simulink model "Q2part5"  (R2018b)
settings: Solver=VariableStepAuto  StartTime=0.0  StopTime=5  RelTol=1e-3
values from neighbouring files (symbols this model uses):
  A = [0           1                 0                          0 ... (first row only)    [Q2.m]
  B1 = [0 1/m1 0 1/m1+1/m2]'    [Q2.m]
  B2 = [0                 0 ... (first row only)    [Q2.m]
  C = [0 0 1 0]    [Q2.m]
  l = L'    [Q2.m]
settings Model: Creator=Asus  LastModifiedBy=Asus

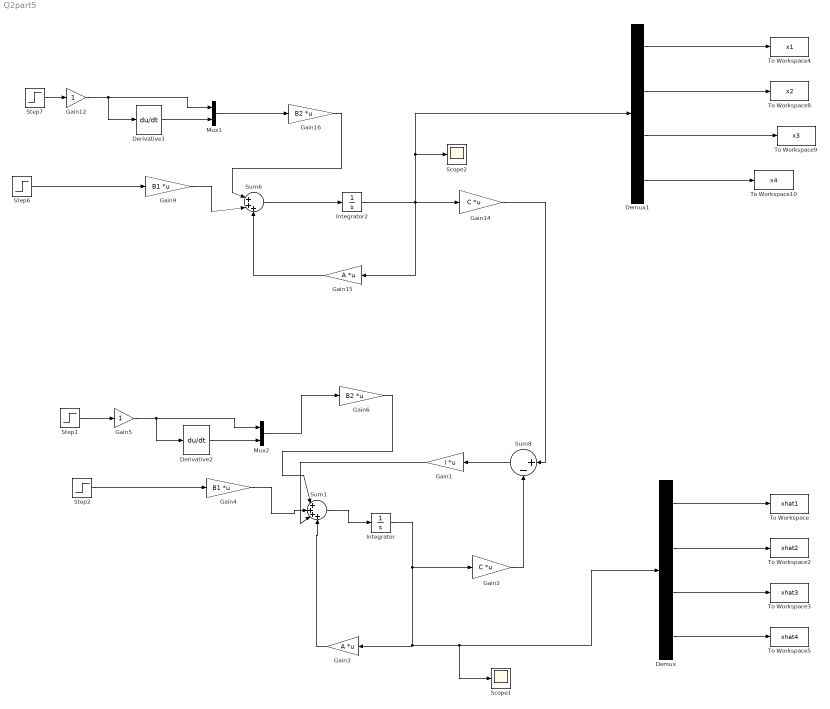
== system Q2part5 ==
  Demux : Demux
  Demux1 : Demux
  Derivative1 : Derivative
  Derivative2 : Derivative
  Gain1 : Gain  Gain=l  Multiplication=Matrix(K*u)
  Gain12 : Gain
  Gain14 : Gain  Gain=C  Multiplication=Matrix(K*u)
  Gain15 : Gain  Gain=A  Multiplication=Matrix(K*u)
  Gain16 : Gain  Gain=B2  Multiplication=Matrix(K*u)
  Gain2 : Gain  Gain=C  Multiplication=Matrix(K*u)
  Gain3 : Gain  Gain=A  Multiplication=Matrix(K*u)
  Gain4 : Gain  Gain=B1  Multiplication=Matrix(K*u)
  Gain5 : Gain
  Gain6 : Gain  Gain=B2  Multiplication=Matrix(K*u)
  Gain9 : Gain  Gain=B1  Multiplication=Matrix(K*u)
  Integrator : Integrator  InitialCondition=[0.5 0 0 0]
  Integrator2 : Integrator
  Mux1 : Mux  Inputs=2
  Mux2 : Mux  Inputs=2
  Scope1 : Scope
  Scope2 : Scope
  Step1 : Step  Time=0  After=0.25  SampleTime=0
  Step2 : Step  Time=0  After=0  SampleTime=0
  Step6 : Step  Time=0  After=0  SampleTime=0
  Step7 : Step  Time=0  After=0.25  SampleTime=0
  Sum1 : Sum  Inputs=|++++
  Sum6 : Sum  Inputs=|+++
  Sum8 : Sum  Inputs=|+-
  To Workspace : ToWorkspace  VariableName=xhat1  SaveFormat=Timeseries  SampleTime=-1
  To Workspace10 : ToWorkspace  VariableName=x4  SaveFormat=Timeseries  SampleTime=-1
  To Workspace2 : ToWorkspace  VariableName=xhat2  SaveFormat=Timeseries  SampleTime=-1
  To Workspace3 : ToWorkspace  VariableName=xhat3  SaveFormat=Timeseries  SampleTime=-1
  To Workspace4 : ToWorkspace  VariableName=x1  SaveFormat=Timeseries  SampleTime=-1
  To Workspace5 : ToWorkspace  VariableName=xhat4  SaveFormat=Timeseries  SampleTime=-1
  To Workspace8 : ToWorkspace  VariableName=x2  SaveFormat=Timeseries  SampleTime=-1
  To Workspace9 : ToWorkspace  VariableName=x3  SaveFormat=Timeseries  SampleTime=-1
  wires:
  Sum1/1 -> Integrator/1
  Gain3/1 -> Sum1/4
  Mux1/1 -> Gain16/1
  Step7/1 -> Gain12/1
  Gain9/1 -> Sum6/2
  Derivative1/1 -> Mux1/2
  Gain16/1 -> Sum6/1
  Gain12/1 -> Derivative1/1, Mux1/1
  Sum6/1 -> Integrator2/1
  Gain15/1 -> Sum6/3
  Gain2/1 -> Sum8/2
  Gain14/1 -> Sum8/1
  Sum8/1 -> Gain1/1
  Step1/1 -> Gain5/1
  Gain5/1 -> Derivative2/1, Mux2/1
  Derivative2/1 -> Mux2/2
  Demux1/2 -> To Workspace8/1
  Demux1/1 -> To Workspace4/1
  Integrator2/1 -> Demux1/1, Scope2/1, Gain15/1, Gain14/1
  Demux1/3 -> To Workspace9/1
  Step6/1 -> Gain9/1
  Gain1/1 -> Sum1/3
  Step2/1 -> Gain4/1
  Gain4/1 -> Sum1/2
  Mux2/1 -> Gain6/1
  Gain6/1 -> Sum1/1
  Integrator/1 -> Scope1/1, Demux/1, Gain3/1, Gain2/1
  Demux/1 -> To Workspace/1
  Demux/2 -> To Workspace2/1
  Demux/3 -> To Workspace3/1
  Demux/4 -> To Workspace5/1
  Demux1/4 -> To Workspace10/1
